simulink model "motor_ideal"  (R2023b)
settings: Solver=VariableStepAuto  StartTime=0.0  StopTime=5.0  RelTol=1e-3
values from neighbouring files (symbols this model uses):
  ke0 = mean(ke)    [caracterizador.m]
  p0 = mean(p)    [caracterizador.m]
  Vref = V(i)    [caracterizador.m]
settings Model: Creator=Matlab  LastModifiedBy=erwinplanck
settings ModelReferenceCC: EnableRefExpFcnMdlSchedulingChecks=on

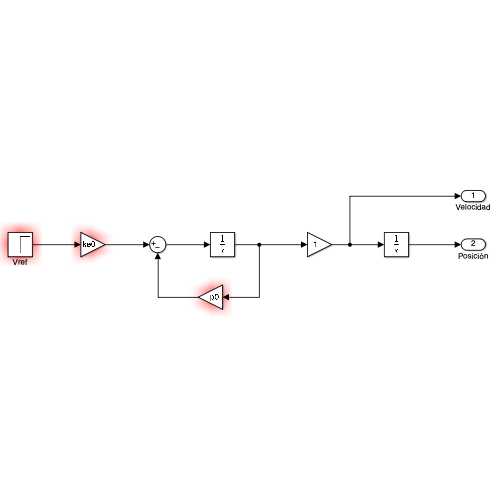
[thumbnail: Simulink's stored preview of the top-level diagram]
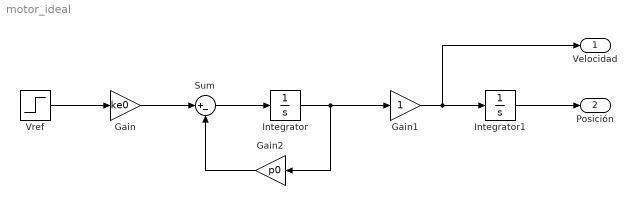
== system motor_ideal ==
  Gain : Gain  Gain=ke0
  Gain1 : Gain
  Gain2 : Gain  Gain=p0
  Integrator : Integrator
  Integrator1 : Integrator
  Sum : Sum  Inputs=|+-
  Vref : Step  After=Vref  SampleTime=0
  Velocidad : Outport
  Posición : Outport  Port=2
  wires:
  Vref/1 -> Gain/1
  Gain/1 -> Sum/1
  Sum/1 -> Integrator/1
  Integrator/1 -> Gain2/1, Gain1/1
  Gain1/1 -> Velocidad/1, Integrator1/1
  Gain2/1 -> Sum/2
  Integrator1/1 -> Posición/1
